simulink model "controlGPI_pos_3dof_sinMI"  (R2023b)
settings: Solver=VariableStepAuto  StartTime=0.0  StopTime=tsim  FixedStep=1e-5  MaxStep=tstep  RelTol=1e-3
undefined symbols (not defined in the file): contr_robot_params, ddq, dq, ndof, NN_Bspline_params, NN_RBF_params, nn_select, Pc, q, q0, q_cero, q_eq, robot_params, t_qeq_init, t_tr_init, t_trtr, tau_L, tau_L_mags, tr_muestra, Wc, Zc
libraries: simulink x2
(part 2 of 2)

== matlab function controlGPI_pos_3dof_sinMI/q to xyz (robot)/q to xyz (referencia) ==
  data: p output size=[3,3]; robot_params input; q input size=[3,1]; dq input size=[3,1]; ddq input size=[3,1]; dp output size=[3,1]; ddp output size=[3,1]
function [p,dp,ddp] = fcn(robot_params,q,dq,ddq)

[p,dp,ddp] = robot_cin.cin_dir_3dof(robot_params,q,dq,ddq);

== matlab function controlGPI_pos_3dof_sinMI/Trayectoria de referencia/xyz to q (referencia) ==
  data: robot_params input; q output size=[3,1]; r input size=[3,1]; dr input size=[3,1]; ddr input size=[3,1]; dq output size=[3,1]; ddq output size=[3,1]
function [q,dq,ddq] = fcn(robot_params,r,dr,ddr)

[q,dq,ddq] = robot_cin.cin_inv_3dof(robot_params,r,dr,ddr);

== matlab function controlGPI_pos_3dof_sinMI/ControladorGPI + NN/Matriz D ==
  data: robot_params input Bus: robot_params_bus; robot_din output Bus: robot_din_bus; q input
function robot_din = fcn(robot_params,q)

robot_din = robot_dinm.din_3dof(robot_params,q,zeros(size(q)));

== matlab function controlGPI_pos_3dof_sinMI/Perfil torque de carga tau_L/If Action Subsystem/Polinomio 7mo orden sen ==
  data: t input; perfil_params input; qpol output; vpol output; apol output; jpol output
function [qpol,vpol,apol,jpol] = fcn(t,perfil_params)

%Trayectoria de referencia

q0 = 0;
q1 = perfil_params.senoidal.amplitud;

% v0 = perfil_params.polinomio7.vel.inicial;
% v1 = perfil_params.polinomio7.vel.final;
% 
% ac0 = perfil_params.polinomio7.acel.inicial;
% ac1 = perfil_params.polinomio7.acel.final;
% 
% j0 = perfil_params.polinomio7.jerk.inicial;
% j1 = perfil_params.polinomio7.jerk.inicial;

if perfil_params.senoidal.tiempo_inicio-1>0
    t0 = perfil_params.senoidal.tiempo_inicio-1;
else
    t0 = 0;
end
t1 = perfil_params.senoidal.tiempo_inicio;

% Coeficientes de un polinomio de 7mo grado
[qpol,vpol,apol,jpol] = pol7(t,q1,q0,t0,t1);

== matlab function controlGPI_pos_3dof_sinMI/Perfil torque de carga tau_L/If Action Subsystem4/Polinomio 7mo orden tau_L ==
  data: t input; perfil_params input; qpol output; vpol output; apol output; jpol output
function [qpol,vpol,apol,jpol] = fcn(t,perfil_params)

%Trayectoria de referencia

q0 = perfil_params.polinomio7.pos.inicial;
q1 = perfil_params.polinomio7.pos.final;

% v0 = perfil_params.polinomio7.vel.inicial;
% v1 = perfil_params.polinomio7.vel.final;
% 
% ac0 = perfil_params.polinomio7.acel.inicial;
% ac1 = perfil_params.polinomio7.acel.final;
% 
% j0 = perfil_params.polinomio7.jerk.inicial;
% j1 = perfil_params.polinomio7.jerk.inicial;

t0 = perfil_params.polinomio7.tiempo.inicial;
t1 = perfil_params.polinomio7.tiempo.final;

% Coeficientes de un polinomio de 7mo grado
[qpol,vpol,apol,jpol] = pol7(t,q0,q1,t0,t1);

== matlab function controlGPI_pos_3dof_sinMI/Perfil torque de carga tau_L/If Action Subsystem7/Trayectoria 15 segmentos ==
  data: t input size=1; q output size=1; perfil_params input
function q = fcn(t,perfil_params)

q0 = perfil_params.tr15segs.pos.inicial;
q1 = perfil_params.tr15segs.pos.final;

t0 = perfil_params.tr15segs.tiempo.inicial;

vel_path = perfil_params.tr15segs.vel_path;
acel_path = perfil_params.tr15segs.acel_path;
snap_path = perfil_params.tr15segs.snap_path;

dist = norm(q1-q0);
num_steps = 1000;




[interq,T] = pol15segs.bounded_tr(dist,num_steps,vel_path,acel_path,snap_path,0);

tstep = T/num_steps;
t1 = t0 + T;
t_tr = (t0:tstep:t1)';


[~,idt] = min(t_tr-t);
dire = (q1 - q0)/dist;
q = q0 + dire*interq(idt);

== matlab function controlGPI_pos_3dof_sinMI/Perfil torque de carga tau_L/If Action Subsystem6/Polinomio 7mo orden timeseries ==
  data: t input; qpol output; vpol output; apol output; jpol output
function [qpol,vpol,apol,jpol] = fcn(t)

q0 = 0;
q1 = 1;

t0 = 0.5;
t1 = 1;

%Trayectoria de referencia

% Coeficientes de un polinomio de 7mo grado
[qpol,vpol,apol,jpol] = pol7(t,q0,q1,t0,t1);

== matlab function controlGPI_pos_3dof_sinMI/Perfil torque de carga tau_L/If Action Subsystem/Senoidal tiempo de inicio ==
  data: t input; tr output; perfil_params input
function tr = fcn(t,perfil_params)

t1 = perfil_params.senoidal.tiempo_inicio;

if t < t1
    tr = 0;
else
    tr = t - t1;
end

== matlab function controlGPI_pos_3dof_sinMI/Perfil torque de carga tau_L/If Action Subsystem5/Tren de esca ==
  data: t input; q output; perfil_params input
function q = fcn(t,perfil_params)

q = Perfil_trayectoria.trEsca(t,perfil_params);

== matlab function controlGPI_pos_3dof_sinMI/Modelo robot manipulador (Dinámica directa)/Dinámica directa ==
  data: robot_params input; q input; ddq output size=[3,1]; dq input size=[3,1]; tau_R input size=[3,1]; tau_L input size=[3,1]
function ddq = fcn(robot_params,q,dq,tau_R,tau_L)

robot_din = robot_dinm.din_3dof(robot_params,q,dq);

D = robot_din.D;
C = robot_din.C;
G = robot_din.G;
g = robot_din.g;

ddq = D^-1*(-C*dq-G*g+(tau_R-tau_L));

== matlab function controlGPI_pos_3dof_sinMI/Norm e_q ==
  data: u input; y output
function y = norm(u)

y = norm(u,2);

== matlab function controlGPI_pos_3dof_sinMI/Trayectoria de referencia/Dinamica inversa (referencia) ==
  data: robot_params input; tau_s output size=[3,1]; q input size=[3,1]; dq input size=[3,1]; ddq input size=[3,1]
function tau_s = fcn(robot_params,q,dq,ddq)

robot_din = robot_dinm.din_3dof(robot_params,q,dq);

D = robot_din.D;
C = robot_din.C;
G = robot_din.G;
g = robot_din.g;

tau_s = D*ddq + C*dq + G*g;

== matlab function controlGPI_pos_3dof_sinMI/ControladorGPI + NN/Ley de control ==
  data: robot_din input; v output size=[3,1]; eqB5 input size=[3,1]; eqB4 input size=[3,1]; eqB3 input size=[3,1]; eqB2 input size=[3,1]; eqB1 input size=[3,1]; tau_R output size=[3,1]
function [v,tau_R] = fcn(robot_din,eqB5,eqB4,eqB3,eqB2,eqB1)

D = robot_din.D;

v = - eqB5 - eqB4 - eqB3 - eqB2 - eqB1;

tau_R = D*v;

== matlab function controlGPI_pos_3dof_sinMI/Trayectoria de referencia/Inicializar posición de robot manipulador/interp_pol7_q_r ==
  data: t input; q_eq input; interp_qpos output; q_cero input; q_tr_init input; t0 input; t1 input; t_trtr input; tr_muestra input; ndof input
function interp_qpos = fcn(t,q_eq,q_cero,q_tr_init,t0,t1,t_trtr,tr_muestra,ndof)

tcero = t0/2 + t1/2;

if t < tcero
    dist1 = norm(zeros(size(q_eq)) - q_eq);
    
    if dist1 > 0
        qpol1 = pol7(t,0,dist1,t0,tcero);
        dire1 = (zeros(size(q_eq)) - q_eq)/dist1;
        
        interp_qpos = q_eq + dire1*qpol1;
    else
        interp_qpos = q_eq;
    end
elseif t >= tcero && t < t1
    dist2 = norm(q_cero - zeros(size(q_eq)));
    if dist2 > 0
        qpol2 = pol7(t,0,dist2,tcero,t1);
        dire2 = (q_cero - zeros(size(q_eq)))/dist2;
    
        interp_qpos =  zeros(size(q_eq)) + dire2*qpol2;
    else
        interp_qpos = zeros(size(q_eq));
    end
elseif t >= t1 && t < t1 + t_trtr
    if (tr_muestra == 1 || ndof ~= 6) && ndof ~= 2
        dist3 = norm(q_tr_init - q_cero);
        if dist3 > 0
            qpol3 = pol7(t,0,dist3,t1,t1 + t_trtr);
            dire3 = (q_tr_init - q_cero)/dist3;
            
            interp_qpos =  q_cero + dire3*qpol3;
        else
            interp_qpos = q_cero;
        end
    else
        interp_qpos = q_tr_init;
    end
elseif t >= t1 + t_trtr
    interp_qpos = q_tr_init;
else
    interp_qpos = q_eq;
end

== matlab function controlGPI_pos_3dof_sinMI/ControladorGPI + NN/Matriz de parámetros B ==
  data: B5 output size=[3,1]; B4 output size=[3,1]; B3 output size=[3,1]; B2 output size=[3,1]; Zc input size=[3,1]; B1 output size=[3,1]; Wc input size=[3,1]; Pc input size=[3,1]
function [B5,B4,B3,B2,B1] = fcn(Zc,Wc,Pc)

B = zeros(3,6);

B(:,1) = Wc.^4.*Pc;
B(:,2) = 4*Wc.^3.*Zc.*Pc + Wc.^4;
B(:,3) = 4*Wc.^3.*Zc + 4*Wc.^2.*Zc.^2.*Pc + 2.*Wc.^2.*Pc;
B(:,4) = 2*Wc.^2 + 4*Wc.^2.*Zc.^2 + 4*Wc.*Zc.*Pc;
B(:,5) = 4*Wc.*Zc + Pc;
% B(:,6) = ones(3,6);

B1 = B(:,1);
B2 = B(:,2);
B3 = B(:,3);
B4 = B(:,4);
B5 = B(:,5);
% B6 = B(:,6);

== matlab function controlGPI_pos_3dof_sinMI/Trayectoria de referencia/q to xyz (referencia) ==
  data: p output size=[3,3]; robot_params input; q input size=[3,1]; dp output; ddp output; dq input; ddq input
function [p,dp,ddp] = fcn(robot_params,q,dq,ddq)

[p,dp,ddp] = robot_cin.cin_dir_3dof(robot_params,q,dq,ddq);
